simulink model "SimulinkAnalysisofCheetahTail"  (R2022a)
settings: Solver=ode4  StartTime=0.0  StopTime=1.5  FixedStep=0.001  RelTol=1e-3
undefined symbols (not defined in the file): B_cg_H, B_con_H, B_con_L, bar_len, cd_table, Cf, cl_table, g, gear_ratio, int_point_bar, int_point_tail, ITail, M_add, M_cg_H, M_cg_L, M_cg_W, Mb, Mm, Mt, psi3, rho, T_cg_H, T_fur_gap, T_length, T_width_major, T_width_minor, th2_initial, torque_constant, uncertainty_Forces, uncertainty_Position, Vf, windspeed
(part 20 of 21)

== matlab function SimulinkAnalysisofCheetahTail/Model/Forces/NonConstraintForceMatrix_tail_3_added ==
  data: B_con_H parameter; B_con_L parameter; M_add parameter; M_cg_H parameter; M_cg_L parameter; M_cg_W parameter; T_fur_gap parameter; T_length parameter; bar_len parameter; psi3 parameter; Q_added_tail_3_drag output; q input; dq input; ddq input
function Q_added_tail_3_drag = NonConstraintForceMatrix_tail_3_added(B_con_H,B_con_L,M_add,M_cg_H,M_cg_L,M_cg_W,T_fur_gap,T_length,bar_len,psi3,q,dq,ddq)
%#codegen
[x,y,z,phi1,th1,psi1,phi2,th2] = deal(q(1),q(2),q(3),q(4),q(5),q(6),q(7),q(8));
[dx,dy,dz,dphi1,dth1,dpsi1,dphi2,dth2] = deal(dq(1),dq(2),dq(3),dq(4),dq(5),dq(6),dq(7),dq(8));
[ddx,ddy,ddz,ddphi1,ddth1,ddpsi1,ddphi2,ddth2] = deal(ddq(1),ddq(2),ddq(3),ddq(4),ddq(5),ddq(6),ddq(7),ddq(8));
%    This function was generated by the Symbolic Math Toolbox version 9.0.
%    19-Feb-2022 13:43:46

t2 = cos(phi1);
t3 = cos(phi2);
t4 = cos(psi1);
t5 = cos(psi3);
t6 = cos(th1);
t7 = cos(th2);
t8 = sin(phi1);
t9 = sin(phi2);
t10 = sin(psi1);
t11 = sin(psi3);
t12 = sin(th1);
t13 = sin(th2);
t14 = M_cg_L+x;
t15 = M_cg_W+y;
t16 = M_cg_H+z;
t17 = B_con_L.*t6;
t18 = B_con_L.*t12;
t19 = t2.*t4;
t20 = t6.*t7;
t21 = t2.*t10;
t22 = t4.*t8;
t23 = t7.*t12;
t24 = t8.*t10;
t25 = t12.*t13;
t26 = B_con_H.*t2.*t6;
t28 = t6.*t14;
t29 = B_con_H.*t2.*t12;
t30 = B_con_H.*t6.*t8;
t33 = t12.*t14;
t37 = t6.*t9.*t13;
t39 = t6.*t10.*t13;
t41 = t8.*t9.*t12;
t44 = t2.*t3.*t6;
t47 = t2.*t6.*t9;
t48 = t3.*t6.*t8;
t50 = t2.*t6.*t13;
t51 = t3.*t6.*t13;
t53 = t4.*t6.*t13;
t56 = t3.*t8.*t12;
t57 = t6.*t8.*t9;
t62 = t2.*t6.*t15;
t64 = t2.*t6.*t16;
t67 = t6.*t8.*t15;
t68 = t2.*t12.*t16;
t69 = t6.*t8.*t16;
t71 = t8.*t12.*t15;
t99 = t5.*t6.*t8.*t13;
t105 = t6.*t8.*t11.*t13;
t27 = t4.*t17;
t31 = t4.*t18;
t32 = t10.*t17;
t34 = t10.*t18;
t35 = t2.*t25;
t36 = t3.*t25;
t38 = t9.*t23;
t40 = t10.*t23;
t42 = t12.*t24;
t43 = t9.*t25;
t45 = t2.*t20;
t46 = t4.*t20;
t49 = t12.*t19;
t52 = t3.*t23;
t54 = t4.*t23;
t55 = t10.*t20;
t58 = t12.*t21;
t59 = t12.*t22;
t60 = B_con_H.*t6.*t19;
t61 = t4.*t28;
t63 = B_con_H.*t6.*t21;
t65 = t4.*t33;
t66 = t10.*t28;
t70 = t10.*t33;
t72 = -t29;
t73 = -t30;
t75 = -t41;
t80 = t3.*t6.*t22;
t81 = t13.*t44;
t84 = t3.*t8.*t20;
t85 = t6.*t13.*t19;
t86 = t4.*t51;
t89 = t3.*t6.*t24;
t90 = t6.*t9.*t22;
t91 = t2.*t37;
t93 = t8.*t9.*t20;
t94 = t6.*t13.*t21;
t96 = t3.*t39;
t97 = t4.*t37;
t100 = t6.*t9.*t24;
t104 = t10.*t37;
t107 = -t53;
t110 = t6.*t16.*t19;
t111 = t6.*t15.*t22;
t112 = t6.*t16.*t21;
t113 = t6.*t15.*t24;
t114 = -t62;
t115 = -t67;
t116 = -t68;
t117 = -t69;
t118 = t3.*t19.*t20;
t119 = t3.*t20.*t21;
t120 = t9.*t19.*t20;
t121 = t9.*t20.*t21;
t127 = -t99;
t132 = t23+t50;
t74 = -t35;
t76 = -t42;
t77 = -t43;
t78 = t3.*t45;
t79 = t3.*t46;
t82 = t2.*t52;
t83 = t9.*t45;
t87 = t3.*t55;
t88 = t9.*t46;
t92 = t2.*t38;
t95 = t4.*t36;
t98 = t9.*t55;
t101 = -t45;
t102 = t10.*t36;
t103 = t4.*t43;
t106 = -t49;
t108 = -t55;
t109 = t10.*t43;
t123 = -t86;
t125 = -t93;
t130 = -t111;
t131 = -t113;
t133 = t21+t59;
t134 = t22+t58;
t135 = -t118;
t136 = -t119;
t143 = t5.*t132;
t147 = t11.*t132;
t151 = t47+t84;
t155 = t52+t81;
t156 = t54+t85;
t157 = t38+t91;
t158 = t40+t94;
t122 = -t78;
t124 = -t87;
t126 = -t98;
t128 = t4.*t77;
t129 = t10.*t77;
t137 = B_con_H.*t133;
t138 = B_con_H.*t134;
t139 = t20+t74;
t140 = t25+t101;
t141 = t19+t76;
t142 = t24+t106;
t144 = t3.*t133;
t145 = t3.*t134;
t146 = t7.*t134;
t148 = t9.*t133;
t149 = t9.*t134;
t150 = t13.*t134;
t159 = t15.*t133;
t160 = t15.*t134;
t161 = t16.*t133;
t162 = t16.*t134;
t168 = t5.*t13.*t133;
t170 = t11.*t13.*t133;
t178 = -t147;
t182 = t44+t125;
t183 = T_fur_gap.*t151;
t184 = T_fur_gap.*t155;
t185 = bar_len.*t151;
t186 = bar_len.*t155;
t193 = t5.*t156;
t194 = t11.*t156;
t195 = t5.*t157;
t196 = t5.*t158;
t197 = t11.*t157;
t198 = t11.*t158;
t220 = (T_length.*t151)./2.0;
t221 = (T_length.*t155)./2.0;
t223 = t37+t56+t92;
t226 = t51+t75+t82;
t227 = t48+t77+t83;
t264 = t90+t95+t135;
t266 = t100+t102+t136;
t152 = B_con_H.*t141;
t153 = B_con_H.*t142;
t154 = -t138;
t163 = t7.*t144;
t164 = t7.*t145;
t165 = t13.*t145;
t166 = t7.*t148;
t167 = t9.*t146;
t169 = t13.*t149;
t171 = t5.*t139;
t172 = t5.*t140;
t173 = t3.*t141;
t174 = t3.*t142;
t175 = t7.*t142;
t176 = t11.*t139;
t177 = t11.*t140;
t179 = t9.*t141;
t180 = t9.*t142;
t181 = t13.*t142;
t187 = t15.*t141;
t188 = t15.*t142;
t189 = -t160;
t190 = t16.*t141;
t191 = t16.*t142;
t192 = -t162;
t205 = t5.*t13.*t141;
t207 = t11.*t13.*t141;
t208 = -t170;
t214 = t5.*t182;
t215 = t11.*t182;
t216 = -t198;
t222 = t39+t146;
t224 = t108+t150;
t225 = t36+t57+t122;
t231 = t5.*t223;
t232 = t11.*t223;
t235 = T_fur_gap.*t226;
t236 = T_fur_gap.*t227;
t237 = bar_len.*t226;
t238 = bar_len.*t227;
t241 = -t5.*(t55-t150);
t244 = -t11.*(t55-t150);
t245 = t5.*t227;
t247 = t11.*t227;
t257 = (T_length.*t226)./2.0;
t258 = (T_length.*t227)./2.0;
t265 = t80+t120+t128;
t267 = t89+t121+t129;
t274 = T_fur_gap.*t264;
t275 = bar_len.*t264;
t276 = T_fur_gap.*t266;
t277 = bar_len.*t266;
t285 = (T_length.*t264)./2.0;
t286 = (T_length.*t266)./2.0;
t353 = t184+t186+t221;
t373 = t73+t114+t117+t183+t185+t220;
t199 = t7.*t173;
t200 = t7.*t174;
t201 = -t163;
t202 = t13.*t174;
t203 = t7.*t179;
t204 = t9.*t175;
t206 = t13.*t180;
t209 = -t171;
t210 = -t173;
t211 = -t177;
t212 = -t187;
t213 = -t188;
t219 = -t207;
t228 = t46+t181;
t229 = t5.*t222;
t230 = t11.*t222;
t233 = T_fur_gap.*t225;
t234 = bar_len.*t225;
t239 = t107+t175;
t246 = t12.*t225;
t249 = t124+t165;
t251 = t126+t169;
t252 = t2.*t6.*t225;
t253 = -t5.*(t53-t175);
t254 = t6.*t8.*t225;
t255 = -t11.*(t53-t175);
t256 = (T_length.*t225)./2.0;
t261 = -T_fur_gap.*(t87-t165);
t262 = -bar_len.*(t87-t165);
t263 = t105+t214;
t268 = -t5.*(t98-t169);
t270 = -t11.*(t98-t169);
t272 = t5.*(t53-t175);
t278 = t127+t215;
t279 = t5.*t267;
t280 = t11.*t267;
t282 = T_length.*(t87-t165).*(-1.0./2.0);
t283 = t5.*t265;
t284 = t11.*t265;
t288 = t166+t174;
t290 = t172+t197;
t298 = -T_fur_gap.*(t163-t180);
t300 = -bar_len.*(t163-t180);
t303 = T_length.*(t163-t180).*(-1.0./2.0);
t304 = t143+t247;
t305 = t96+t164+t179;
t306 = t176+t231;
t310 = t178+t245;
t328 = -t12.*(t147-t245);
t336 = -t2.*t6.*(t147-t245);
t337 = -t6.*t8.*(t147-t245);
t343 = t2.*t6.*(t147-t245);
t367 = t236+t238+t258;
t368 = t225.*t353;
t385 = -t353.*(t147-t245);
t386 = t353.*(t147-t245);
t388 = -t225.*(t30+t62+t69-t183-t185-t220);
t391 = t17+t28+t71+t72+t116+t235+t237+t257;
t397 = (t147-t245).*(t30+t62+t69-t183-t185-t220);
t407 = t31+t60+t65+t110+t130+t274+t275+t285;
t408 = t34+t63+t70+t112+t131+t276+t277+t286;
t217 = -t199;
t218 = -t204;
t240 = t5.*t228;
t242 = t11.*t228;
t243 = -t229;
t248 = t79+t202;
t250 = t88+t206;
t271 = -t252;
t287 = t145+t203;
t289 = -t283;
t292 = t180+t201;
t294 = t5.*t288;
t296 = t11.*t288;
t301 = t195+t211;
t307 = T_fur_gap.*t305;
t308 = bar_len.*t305;
t309 = t123+t148+t200;
t312 = t209+t232;
t313 = t104+t167+t210;
t314 = t12.*t304;
t321 = (T_length.*t305)./2.0;
t322 = t2.*t6.*t304;
t323 = t6.*t8.*t304;
t324 = t6.*t10.*t305;
t344 = t193+t284;
t345 = t196+t280;
t347 = t216+t279;
t349 = t134.*t305;
t350 = t230+t268;
t355 = t141.*t305;
t383 = t261+t262+t282;
t384 = t304.*t353;
t387 = t225.*t367;
t390 = t18+t26+t33+t64+t115+t233+t234+t256;
t392 = t304.*t367;
t393 = -t304.*(t30+t62+t69-t183-t185-t220);
t395 = -t367.*(t147-t245);
t399 = -t397;
t402 = -t305.*(T_fur_gap.*(t87-t165)+(T_length.*(t87-t165))./2.0+bar_len.*(t87-t165));
t406 = t305.*(T_fur_gap.*(t87-t165)+(T_length.*(t87-t165))./2.0+bar_len.*(t87-t165));
t411 = t225.*t391;
t432 = t304.*t391;
t433 = -t391.*(t147-t245);
t435 = t137+t161+t213+t298+t300+t303;
t441 = t305.*t408;
t259 = T_fur_gap.*t248;
t260 = bar_len.*t248;
t269 = t11.*t250;
t273 = t5.*t250;
t281 = (T_length.*t248)./2.0;
t291 = t149+t217;
t293 = t5.*t287;
t295 = t11.*t287;
t311 = t97+t144+t218;
t315 = T_fur_gap.*t309;
t316 = bar_len.*t309;
t319 = T_fur_gap.*t313;
t320 = bar_len.*t313;
t326 = t5.*t313;
t329 = t11.*t313;
t332 = (T_length.*t309)./2.0;
t334 = (T_length.*t313)./2.0;
t335 = t4.*t6.*t309;
t338 = -t323;
t346 = t194+t289;
t348 = t168+t296;
t351 = t208+t294;
t354 = t133.*t309;
t356 = t243+t270;
t358 = t142.*t309;
t389 = -t387;
t396 = -t392;
t400 = t151.*t390;
t401 = t155.*t390;
t403 = t226.*t390;
t404 = t227.*t390;
t412 = t5.*t225.*t390;
t413 = t11.*t225.*t390;
t417 = t263.*t390;
t419 = -t390.*(t99-t215);
t425 = t290.*t390;
t427 = -t390.*(t177-t195);
t429 = t306.*t390;
t430 = -t390.*(t171-t232);
t434 = -t432;
t442 = -t441;
t443 = t309.*t407;
t447 = t32+t66+t154+t192+t212+t307+t308+t321;
t452 = -t309.*(-t137-t161+t188+T_fur_gap.*(t163-t180)+(T_length.*(t163-t180))./2.0+bar_len.*(t163-t180));
t455 = t309.*(-t137-t161+t188+T_fur_gap.*(t163-t180)+(T_length.*(t163-t180))./2.0+bar_len.*(t163-t180));
t297 = T_fur_gap.*t291;
t299 = bar_len.*t291;
t302 = (T_length.*t291)./2.0;
t317 = T_fur_gap.*t311;
t318 = bar_len.*t311;
t325 = t5.*t311;
t327 = t11.*t311;
t330 = -t315;
t331 = -t316;
t333 = (T_length.*t311)./2.0;
t339 = -t326;
t341 = -t332;
t342 = -t335;
t352 = t205+t295;
t357 = t219+t293;
t359 = t255+t273;
t360 = t269+t272;
t362 = t241+t329;
t366 = t6.*t10.*(t329-t5.*(t55-t150));
t371 = -t6.*t10.*(t326+t11.*(t55-t150));
t375 = t134.*(t329-t5.*(t55-t150));
t378 = t141.*(t329-t5.*(t55-t150));
t379 = -t134.*(t326+t11.*(t55-t150));
t381 = -t141.*(t326+t11.*(t55-t150));
t382 = t259+t260+t281;
t409 = -t404;
t414 = -t412;
t415 = t319+t320+t334;
t418 = t254+t354+t355;
t420 = -t417;
t422 = t271+t349+t358;
t428 = -t425;
t431 = -t429;
t438 = -(t329-t5.*(t55-t150)).*(T_fur_gap.*(t87-t165)+(T_length.*(t87-t165))./2.0+bar_len.*(t87-t165));
t440 = (t326+t11.*(t55-t150)).*(T_fur_gap.*(t87-t165)+(T_length.*(t87-t165))./2.0+bar_len.*(t87-t165));
t458 = t408.*(t329-t5.*(t55-t150));
t460 = -t408.*(t326+t11.*(t55-t150));
t464 = t408.*(t326+t11.*(t55-t150));
t477 = -t447.*(t87-t165);
t478 = t447.*(t87-t165);
t479 = t266.*t447;
t484 = t291.*t447;
t492 = t5.*t305.*t447;
t493 = t11.*t305.*t447;
t494 = t313.*t447;
t497 = t345.*t447;
t500 = -t447.*(t198-t279);
t502 = t447.*(t198-t279);
t503 = t350.*t447;
t506 = -t447.*(t229+t11.*(t98-t169));
t508 = -t447.*(t207-t293);
t340 = -t327;
t361 = t242+t325;
t364 = t244+t339;
t372 = -t366;
t394 = t246+t324+t342;
t405 = t309.*t382;
t416 = t317+t318+t333;
t421 = ddy.*t418;
t423 = ddz.*t422;
t437 = t152+t189+t190+t297+t299+t302;
t444 = t305.*t415;
t448 = t27+t61+t153+t159+t191+t330+t331+t341;
t461 = -t458;
t465 = t415.*(t329-t5.*(t55-t150));
t467 = -t415.*(t326+t11.*(t55-t150));
t469 = t415.*(t326+t11.*(t55-t150));
t481 = -t479;
t486 = -t484;
t495 = -t492;
t504 = t352.*t447;
t507 = -t503;
t363 = t240+t340;
t365 = t4.*t6.*t361;
t374 = t133.*t361;
t376 = t142.*t361;
t398 = ddx.*t394;
t410 = -t405;
t424 = -t421;
t426 = -t423;
t436 = t361.*t382;
t445 = t309.*t416;
t453 = t305.*t437;
t459 = t361.*t407;
t463 = t361.*t416;
t468 = -t465;
t482 = t248.*t448;
t483 = t264.*t448;
t487 = -t361.*(-t137-t161+t188+T_fur_gap.*(t163-t180)+(T_length.*(t163-t180))./2.0+bar_len.*(t163-t180));
t489 = t437.*(t329-t5.*(t55-t150));
t490 = -t437.*(t326+t11.*(t55-t150));
t491 = -t448.*(t163-t180);
t496 = t311.*t448;
t498 = t5.*t309.*t448;
t499 = t11.*t309.*t448;
t505 = t344.*t448;
t509 = -t504;
t510 = t346.*t448;
t511 = t348.*t448;
t512 = -t448.*(t170-t294);
t513 = t448.*(t170-t294);
t514 = t359.*t448;
t515 = t360.*t448;
t369 = t4.*t6.*t363;
t370 = -t365;
t377 = t133.*t363;
t380 = t142.*t363;
t439 = t363.*t382;
t446 = -t445;
t454 = -ddx.*(t365+t12.*(t147-t245)+t6.*t10.*(t326+t11.*(t55-t150)));
t456 = -t453;
t457 = ddx.*(t365+t12.*(t147-t245)+t6.*t10.*(t326+t11.*(t55-t150)));
t462 = t363.*t407;
t466 = t363.*t416;
Q_added_tail_3_drag = ft_1({M_add,T_fur_gap,T_length,bar_len,ddphi1,ddphi2,ddth1,ddth2,ddx,ddy,ddz,t10,t11,t12,t132,t133,t134,t137,t141,t142,t147,t150,t161,t163,t165,t169,t171,t180,t183,t185,t188,t2,t207,t215,t220,t225,t227,t228,t229,t232,t245,t293,t30,t304,t305,t309,t311,t313,t314,t322,t326,t328,t329,t337,t338,t343,t353,t361,t363,t367,t368,t369,t370,t371,t372,t374,t375,t376,t377,t378,t379,t380,t381,t382,t384,t386,t387,t388,t389,t390,t391,t392,t393,t395,t396,t397,t398,t399,t4,t400,t401,t403,t404,t406,t407,t408,t409,t410,t411,t413,t414,t415,t416,t417,t419,t420,t424,t425,t426,t427,t428,t430,t431,t432,t433,t434,t436,t437,t438,t439,t440,t442,t443,t444,t445,t446,t447,t448,t452,t453,t454,t455,t456,t457,t458,t459,t461,t462,t463,t464,t465,t466,t468,t469,t478,t481,t482,t483,t484,t486,t487,t489,t490,t491,t493,t494,t495,t496,t497,t498,t499,t5,t502,t504,t505,t506,t507,t508,t509,t510,t511,t512,t513,t514,t515,t55,t6,t62,t69,t8,t87,t98,t99});
end
function Q_added_tail_3_drag = ft_1(ct)
M_add = ct{1};
T_fur_gap = ct{2};
T_length = ct{3};
bar_len = ct{4};
ddphi1 = ct{5};
ddphi2 = ct{6};
ddth1 = ct{7};
ddth2 = ct{8};
ddx = ct{9};
ddy = ct{10};
ddz = ct{11};
t10 = ct{12};
t11 = ct{13};
t12 = ct{14};
t132 = ct{15};
t133 = ct{16};
t134 = ct{17};
t137 = ct{18};
t141 = ct{19};
t142 = ct{20};
t147 = ct{21};
t150 = ct{22};
t161 = ct{23};
t163 = ct{24};
t165 = ct{25};
t169 = ct{26};
t171 = ct{27};
t180 = ct{28};
t183 = ct{29};
t185 = ct{30};
t188 = ct{31};
t2 = ct{32};
t207 = ct{33};
t215 = ct{34};
t220 = ct{35};
t225 = ct{36};
t227 = ct{37};
t228 = ct{38};
t229 = ct{39};
t232 = ct{40};
t245 = ct{41};
t293 = ct{42};
t30 = ct{43};
t304 = ct{44};
t305 = ct{45};
t309 = ct{46};
t311 = ct{47};
t313 = ct{48};
t314 = ct{49};
t322 = ct{50};
t326 = ct{51};
t328 = ct{52};
t329 = ct{53};
t337 = ct{54};
t338 = ct{55};
t343 = ct{56};
t353 = ct{57};
t361 = ct{58};
t363 = ct{59};
t367 = ct{60};
t368 = ct{61};
t369 = ct{62};
t370 = ct{63};
t371 = ct{64};
t372 = ct{65};
t374 = ct{66};
t375 = ct{67};
t376 = ct{68};
t377 = ct{69};
t378 = ct{70};
t379 = ct{71};
t380 = ct{72};
t381 = ct{73};
t382 = ct{74};
t384 = ct{75};
t386 = ct{76};
t387 = ct{77};
t388 = ct{78};
t389 = ct{79};
t390 = ct{80};
t391 = ct{81};
t392 = ct{82};
t393 = ct{83};
t395 = ct{84};
t396 = ct{85};
t397 = ct{86};
t398 = ct{87};
t399 = ct{88};
t4 = ct{89};
t400 = ct{90};
t401 = ct{91};
t403 = ct{92};
t404 = ct{93};
t406 = ct{94};
t407 = ct{95};
t408 = ct{96};
t409 = ct{97};
t410 = ct{98};
t411 = ct{99};
t413 = ct{100};
t414 = ct{101};
t415 = ct{102};
t416 = ct{103};
t417 = ct{104};
t419 = ct{105};
t420 = ct{106};
t424 = ct{107};
t425 = ct{108};
t426 = ct{109};
t427 = ct{110};
t428 = ct{111};
t430 = ct{112};
t431 = ct{113};
t432 = ct{114};
t433 = ct{115};
t434 = ct{116};
t436 = ct{117};
t437 = ct{118};
t438 = ct{119};
t439 = ct{120};
t440 = ct{121};
t442 = ct{122};
t443 = ct{123};
t444 = ct{124};
t445 = ct{125};
t446 = ct{126};
t447 = ct{127};
t448 = ct{128};
t452 = ct{129};
t453 = ct{130};
t454 = ct{131};
t455 = ct{132};
t456 = ct{133};
t457 = ct{134};
t458 = ct{135};
t459 = ct{136};
t461 = ct{137};
t462 = ct{138};
t463 = ct{139};
t464 = ct{140};
t465 = ct{141};
t466 = ct{142};
t468 = ct{143};
t469 = ct{144};
t478 = ct{145};
t481 = ct{146};
t482 = ct{147};
t483 = ct{148};
t484 = ct{149};
t486 = ct{150};
t487 = ct{151};
t489 = ct{152};
t490 = ct{153};
t491 = ct{154};
t493 = ct{155};
t494 = ct{156};
t495 = ct{157};
t496 = ct{158};
t497 = ct{159};
t498 = ct{160};
t499 = ct{161};
t5 = ct{162};
t502 = ct{163};
t504 = ct{164};
t505 = ct{165};
t506 = ct{166};
t507 = ct{167};
t508 = ct{168};
t509 = ct{169};
t510 = ct{170};
t511 = ct{171};
t512 = ct{172};
t513 = ct{173};
t514 = ct{174};
t515 = ct{175};
t55 = ct{176};
t6 = ct{177};
t62 = ct{178};
t69 = ct{179};
t8 = ct{180};
t87 = ct{181};
t98 = ct{182};
t99 = ct{183};
t471 = t337+t374+t381;
t474 = -ddy.*(-t374+t141.*(t326+t11.*(t55-t150))+t6.*t8.*(t147-t245));
t476 = t343+t376+t379;
t485 = -t483;
t488 = -t363.*(-t137-t161+t188+T_fur_gap.*(t163-t180)+(T_length.*(t163-t180))./2.0+bar_len.*(t163-t180));
t501 = -t499;
t516 = -t515;
t517 = t368+t401+t406+t410+t478+t482;
t522 = t386+t427+t436+t440+t507+t514;
t524 = -ddphi2.*(t387+t404-t444+t445-t494-t496);
t527 = ddphi2.*(t387+t404-t444+t445-t494-t496);
t529 = -ddphi1.*(-t400+t452+t453+t484+t225.*(t30+t62+t69-t183-t185-t220)+t448.*(t163-t180));
t532 = t395+t414+t463+t469+t495+t498;
t539 = t431+t433+t459+t464+t502+t510;
t543 = -ddphi1.*(-t489+t504-t511+t304.*(t30+t62+t69-t183-t185-t220)+t363.*(-t137-t161+t188+T_fur_gap.*(t163-t180)+(T_length.*(t163-t180))./2.0+bar_len.*(t163-t180))+t390.*(t99-t215));
t544 = t399+t420+t487+t490+t508+t513;
t545 = -ddphi1.*(t397+t417+t512+t437.*(t326+t11.*(t55-t150))+t361.*(-t137-t161+t188+T_fur_gap.*(t163-t180)+(T_length.*(t163-t180))./2.0+bar_len.*(t163-t180))+t447.*(t207-t293));
t449 = t314+t369+t372;
t451 = t328+t370+t371;
t470 = t322+t375+t380;
t472 = t338+t377+t378;
t480 = ddz.*t476;
t518 = ddth2.*t517;
t519 = t403+t411+t442+t443+t481+t485;
t521 = t389+t409+t444+t446+t494+t496;
t523 = t384+t428+t438+t439+t506+t516;
t525 = ddth2.*t522;
t526 = -ddth2.*(-t384+t425-t439+t515+t447.*(t229+t11.*(t98-t169))+(t329-t5.*(t55-t150)).*(T_fur_gap.*(t87-t165)+(T_length.*(t87-t165))./2.0+bar_len.*(t87-t165)));
t528 = t388+t400+t455+t456+t486+t491;
t530 = t396+t413+t466+t468+t493+t501;
t531 = -ddphi2.*(t392-t413+t465-t466-t493+t499);
t533 = ddphi2.*(t392-t413+t465-t466-t493+t499);
t534 = ddphi2.*t532;
t536 = t430+t434+t461+t462+t497+t505;
t537 = -ddth1.*(t432+t458-t462-t497-t505+t390.*(t171-t232));
t538 = ddth1.*(t432+t458-t462-t497-t505+t390.*(t171-t232));
t540 = ddth1.*t539;
t542 = t393+t419+t488+t489+t509+t511;
t450 = ddx.*t449;
t473 = ddz.*t470;
t475 = ddy.*t472;
t520 = ddth1.*t519;
t535 = -t534;
t541 = -t540;
t557 = -M_add.*t227.*(t454-t480-t525+t534+t540+ddy.*(-t374+t141.*(t326+t11.*(t55-t150))+t6.*t8.*(t147-t245))+ddphi1.*(t397+t417+t512+t437.*(t326+t11.*(t55-t150))+t361.*(-t137-t161+t188+T_fur_gap.*(t163-t180)+(T_length.*(t163-t180))./2.0+bar_len.*(t163-t180))+t447.*(t207-t293)));
t558 = M_add.*t227.*(t454-t480-t525+t534+t540+ddy.*(-t374+t141.*(t326+t11.*(t55-t150))+t6.*t8.*(t147-t245))+ddphi1.*(t397+t417+t512+t437.*(t326+t11.*(t55-t150))+t361.*(-t137-t161+t188+T_fur_gap.*(t163-t180)+(T_length.*(t163-t180))./2.0+bar_len.*(t163-t180))+t447.*(t207-t293)));
t559 = -M_add.*t311.*(t454-t480-t525+t534+t540+ddy.*(-t374+t141.*(t326+t11.*(t55-t150))+t6.*t8.*(t147-t245))+ddphi1.*(t397+t417+t512+t437.*(t326+t11.*(t55-t150))+t361.*(-t137-t161+t188+T_fur_gap.*(t163-t180)+(T_length.*(t163-t180))./2.0+bar_len.*(t163-t180))+t447.*(t207-t293)));
t560 = -M_add.*t313.*(t454-t480-t525+t534+t540+ddy.*(-t374+t141.*(t326+t11.*(t55-t150))+t6.*t8.*(t147-t245))+ddphi1.*(t397+t417+t512+t437.*(t326+t11.*(t55-t150))+t361.*(-t137-t161+t188+T_fur_gap.*(t163-t180)+(T_length.*(t163-t180))./2.0+bar_len.*(t163-t180))+t447.*(t207-t293)));
t546 = t398+t424+t426+t518+t520+t527+t529;
t551 = t450+t473+t475+t526+t533+t538+t543;
t553 = t457+t474+t480+t525+t535+t541+t545;
t547 = M_add.*t225.*t546;
t548 = M_add.*t305.*t546;
t549 = M_add.*t309.*t546;
t552 = M_add.*t132.*t551;
t554 = M_add.*t228.*t551;
t555 = -M_add.*t551.*(t55-t150);
t556 = M_add.*t551.*(t55-t150);
t550 = -t549;
t561 = t547+t552+t558;
t562 = t548+t556+t560;
t563 = t550+t554+t559;
mt1 = [-t12.*t561-t6.*t10.*t562+t4.*t6.*(t549-t554+M_add.*t311.*(t454-t480-t525+t534+t540+ddy.*(-t374+t141.*(t326+t11.*(t55-t150))+t6.*t8.*(t147-t245))+ddphi1.*(t397+t417+t512+t437.*(t326+t11.*(t55-t150))+t361.*(-t137-t161+t188+T_fur_gap.*(t163-t180)+(T_length.*(t163-t180))./2.0+bar_len.*(t163-t180))+t447.*(t207-t293))))];
mt2 = [t141.*t562+t133.*(t549-t554+M_add.*t311.*(t454-t480-t525+t534+t540+ddy.*(-t374+t141.*(t326+t11.*(t55-t150))+t6.*t8.*(t147-t245))+ddphi1.*(t397+t417+t512+t437.*(t326+t11.*(t55-t150))+t361.*(-t137-t161+t188+T_fur_gap.*(t163-t180)+(T_length.*(t163-t180))./2.0+bar_len.*(t163-t180))+t447.*(t207-t293))))+t6.*t8.*t561];
mt3 = [t134.*t562+t142.*(t549-t554+M_add.*t311.*(t454-t480-t525+t534+t540+ddy.*(-t374+t141.*(t326+t11.*(t55-t150))+t6.*t8.*(t147-t245))+ddphi1.*(t397+t417+t512+t437.*(t326+t11.*(t55-t150))+t361.*(-t137-t161+t188+T_fur_gap.*(t163-t180)+(T_length.*(t163-t180))./2.0+bar_len.*(t163-t180))+t447.*(t207-t293))))-t2.*t6.*t561];
mt4 = [t561.*(t30+t62+t69-t183-t185-t220)+t437.*t562-(t549-t554+M_add.*t311.*(t454-t480-t525+t534+t540+ddy.*(-t374+t141.*(t326+t11.*(t55-t150))+t6.*t8.*(t147-t245))+ddphi1.*(t397+t417+t512+t437.*(t326+t11.*(t55-t150))+t361.*(-t137-t161+t188+T_fur_gap.*(t163-t180)+(T_length.*(t163-t180))./2.0+bar_len.*(t163-t180))+t447.*(t207-t293)))).*(-t137-t161+t188+T_fur_gap.*(t163-t180)+(T_length.*(t163-t180))./2.0+bar_len.*(t163-t180))];
mt5 = [-t391.*t561+t408.*t562-t407.*(t549-t554+M_add.*t311.*(t454-t480-t525+t534+t540+ddy.*(-t374+t141.*(t326+t11.*(t55-t150))+t6.*t8.*(t147-t245))+ddphi1.*(t397+t417+t512+t437.*(t326+t11.*(t55-t150))+t361.*(-t137-t161+t188+T_fur_gap.*(t163-t180)+(T_length.*(t163-t180))./2.0+bar_len.*(t163-t180))+t447.*(t207-t293))))];
mt6 = [-t448.*t562-t447.*(t549-t554+M_add.*t311.*(t454-t480-t525+t534+t540+ddy.*(-t374+t141.*(t326+t11.*(t55-t150))+t6.*t8.*(t147-t245))+ddphi1.*(t397+t417+t512+t437.*(t326+t11.*(t55-t150))+t361.*(-t137-t161+t188+T_fur_gap.*(t163-t180)+(T_length.*(t163-t180))./2.0+bar_len.*(t163-t180))+t447.*(t207-t293))))];
mt7 = [-t367.*t561+t415.*t562-t416.*(t549-t554+M_add.*t311.*(t454-t480-t525+t534+t540+ddy.*(-t374+t141.*(t326+t11.*(t55-t150))+t6.*t8.*(t147-t245))+ddphi1.*(t397+t417+t512+t437.*(t326+t11.*(t55-t150))+t361.*(-t137-t161+t188+T_fur_gap.*(t163-t180)+(T_length.*(t163-t180))./2.0+bar_len.*(t163-t180))+t447.*(t207-t293))))];
mt8 = [-t353.*t561-t562.*(T_fur_gap.*(t87-t165)+(T_length.*(t87-t165))./2.0+bar_len.*(t87-t165))+t382.*(t549-t554+M_add.*t311.*(t454-t480-t525+t534+t540+ddy.*(-t374+t141.*(t326+t11.*(t55-t150))+t6.*t8.*(t147-t245))+ddphi1.*(t397+t417+t512+t437.*(t326+t11.*(t55-t150))+t361.*(-t137-t161+t188+T_fur_gap.*(t163-t180)+(T_length.*(t163-t180))./2.0+bar_len.*(t163-t180))+t447.*(t207-t293))))];
Q_added_tail_3_drag = [mt1;mt2;mt3;mt4;mt5;mt6;mt7;mt8];
end

== matlab function SimulinkAnalysisofCheetahTail/Model/Forces/NonConstraintForceMatrix_tail_4_added ==
  data: B_con_H parameter; B_con_L parameter; M_add parameter; M_cg_H parameter; M_cg_L parameter; M_cg_W parameter; T_fur_gap parameter; T_length parameter; bar_len parameter; psi3 parameter; Q_added_tail_4_drag output; q input; dq input; ddq input
function Q_added_tail_4_drag = NonConstraintForceMatrix_tail_4_added(B_con_H,B_con_L,M_add,M_cg_H,M_cg_L,M_cg_W,T_fur_gap,T_length,bar_len,psi3,q,dq,ddq)
%#codegen
[x,y,z,phi1,th1,psi1,phi2,th2] = deal(q(1),q(2),q(3),q(4),q(5),q(6),q(7),q(8));
[dx,dy,dz,dphi1,dth1,dpsi1,dphi2,dth2] = deal(dq(1),dq(2),dq(3),dq(4),dq(5),dq(6),dq(7),dq(8));
[ddx,ddy,ddz,ddphi1,ddth1,ddpsi1,ddphi2,ddth2] = deal(ddq(1),ddq(2),ddq(3),ddq(4),ddq(5),ddq(6),ddq(7),ddq(8));
%    This function was generated by the Symbolic Math Toolbox version 9.0.
%    19-Feb-2022 13:44:13

t2 = cos(phi1);
t3 = cos(phi2);
t4 = cos(psi1);
t5 = cos(psi3);
t6 = cos(th1);
t7 = cos(th2);
t8 = sin(phi1);
t9 = sin(phi2);
t10 = sin(psi1);
t11 = sin(psi3);
t12 = sin(th1);
t13 = sin(th2);
t14 = M_cg_L+x;
t15 = M_cg_W+y;
t16 = M_cg_H+z;
t17 = B_con_L.*t6;
t18 = B_con_L.*t12;
t19 = t2.*t4;
t20 = t6.*t7;
t21 = t2.*t10;
t22 = t4.*t8;
t23 = t7.*t12;
t24 = t8.*t10;
t25 = t12.*t13;
t26 = B_con_H.*t2.*t6;
t28 = t6.*t14;
t29 = B_con_H.*t2.*t12;
t30 = B_con_H.*t6.*t8;
t33 = t12.*t14;
t37 = t6.*t9.*t13;
t39 = t6.*t10.*t13;
t41 = t8.*t9.*t12;
t44 = t2.*t3.*t6;
t47 = t2.*t6.*t9;
t48 = t3.*t6.*t8;
t50 = t2.*t6.*t13;
t51 = t3.*t6.*t13;
t53 = t4.*t6.*t13;
t56 = t3.*t8.*t12;
t57 = t6.*t8.*t9;
t62 = t2.*t6.*t15;
t64 = t2.*t6.*t16;
t67 = t6.*t8.*t15;
t68 = t2.*t12.*t16;
t69 = t6.*t8.*t16;
t71 = t8.*t12.*t15;
t99 = t5.*t6.*t8.*t13;
t105 = t6.*t8.*t11.*t13;
t27 = t4.*t17;
t31 = t4.*t18;
t32 = t10.*t17;
t34 = t10.*t18;
t35 = t2.*t25;
t36 = t3.*t25;
t38 = t9.*t23;
t40 = t10.*t23;
t42 = t12.*t24;
t43 = t9.*t25;
t45 = t2.*t20;
t46 = t4.*t20;
t49 = t12.*t19;
t52 = t3.*t23;
t54 = t4.*t23;
t55 = t10.*t20;
t58 = t12.*t21;
t59 = t12.*t22;
t60 = B_con_H.*t6.*t19;
t61 = t4.*t28;
t63 = B_con_H.*t6.*t21;
t65 = t4.*t33;
t66 = t10.*t28;
t70 = t10.*t33;
t72 = -t29;
t73 = -t30;
t75 = -t41;
t80 = t3.*t6.*t22;
t81 = t13.*t44;
t84 = t3.*t8.*t20;
t85 = t6.*t13.*t19;
t86 = t4.*t51;
t89 = t3.*t6.*t24;
t90 = t6.*t9.*t22;
t91 = t2.*t37;
t93 = t8.*t9.*t20;
t94 = t6.*t13.*t21;
t96 = t3.*t39;
t97 = t4.*t37;
t100 = t6.*t9.*t24;
t104 = t10.*t37;
t107 = -t53;
t110 = t6.*t16.*t19;
t111 = t6.*t15.*t22;
t112 = t6.*t16.*t21;
t113 = t6.*t15.*t24;
t114 = -t62;
t115 = -t67;
t116 = -t68;
t117 = -t69;
t118 = t3.*t19.*t20;
t119 = t3.*t20.*t21;
t120 = t9.*t19.*t20;
t121 = t9.*t20.*t21;
t127 = -t99;
t132 = t23+t50;
t74 = -t35;
t76 = -t42;
t77 = -t43;
t78 = t3.*t45;
t79 = t3.*t46;
t82 = t2.*t52;
t83 = t9.*t45;
t87 = t3.*t55;
t88 = t9.*t46;
t92 = t2.*t38;
t95 = t4.*t36;
t98 = t9.*t55;
t101 = -t45;
t102 = t10.*t36;
t103 = t4.*t43;
t106 = -t49;
t108 = -t55;
t109 = t10.*t43;
t123 = -t86;
t125 = -t93;
t130 = -t111;
t131 = -t113;
t133 = t21+t59;
t134 = t22+t58;
t135 = -t118;
t136 = -t119;
t143 = t5.*t132;
t147 = t11.*t132;
t151 = t47+t84;
t155 = t52+t81;
t156 = t54+t85;
t157 = t38+t91;
t158 = t40+t94;
t122 = -t78;
t124 = -t87;
t126 = -t98;
t128 = t4.*t77;
t129 = t10.*t77;
t137 = B_con_H.*t133;
t138 = B_con_H.*t134;
t139 = t20+t74;
t140 = t25+t101;
t141 = t19+t76;
t142 = t24+t106;
t144 = t3.*t133;
t145 = t3.*t134;
t146 = t7.*t134;
t148 = t9.*t133;
t149 = t9.*t134;
t150 = t13.*t134;
t159 = t15.*t133;
t160 = t15.*t134;
t161 = t16.*t133;
t162 = t16.*t134;
t168 = t5.*t13.*t133;
t170 = t11.*t13.*t133;
t178 = -t147;
t182 = t44+t125;
t183 = T_fur_gap.*t151;
t184 = T_fur_gap.*t155;
t185 = bar_len.*t151;
t186 = bar_len.*t155;
t193 = t5.*t156;
t194 = t11.*t156;
t195 = t5.*t157;
t196 = t5.*t158;
t197 = t11.*t157;
t198 = t11.*t158;
t220 = T_length.*t151.*(7.0./1.0e+1);
t221 = T_length.*t155.*(7.0./1.0e+1);
t223 = t37+t56+t92;
t226 = t51+t75+t82;
t227 = t48+t77+t83;
t261 = t90+t95+t135;
t263 = t100+t102+t136;
t152 = B_con_H.*t141;
t153 = B_con_H.*t142;
t154 = -t138;
t163 = t7.*t144;
t164 = t7.*t145;
t165 = t13.*t145;
t166 = t7.*t148;
t167 = t9.*t146;
t169 = t13.*t149;
t171 = t5.*t139;
t172 = t5.*t140;
t173 = t3.*t141;
t174 = t3.*t142;
t175 = t7.*t142;
t176 = t11.*t139;
t177 = t11.*t140;
t179 = t9.*t141;
t180 = t9.*t142;
t181 = t13.*t142;
t187 = t15.*t141;
t188 = t15.*t142;
t189 = -t160;
t190 = t16.*t141;
t191 = t16.*t142;
t192 = -t162;
t205 = t5.*t13.*t141;
t207 = t11.*t13.*t141;
t208 = -t170;
t214 = t5.*t182;
t215 = t11.*t182;
t216 = -t198;
t222 = t39+t146;
t224 = t108+t150;
t225 = t36+t57+t122;
t231 = t5.*t223;
t232 = t11.*t223;
t235 = T_fur_gap.*t226;
t236 = T_fur_gap.*t227;
t237 = bar_len.*t226;
t238 = bar_len.*t227;
t241 = -t5.*(t55-t150);
t244 = -t11.*(t55-t150);
t245 = t5.*t227;
t247 = t11.*t227;
t262 = t80+t120+t128;
t265 = t89+t121+t129;
t266 = T_length.*t226.*(7.0./1.0e+1);
t267 = T_length.*t227.*(7.0./1.0e+1);
t274 = T_fur_gap.*t261;
t275 = bar_len.*t261;
t276 = T_fur_gap.*t263;
t277 = bar_len.*t263;
t288 = T_length.*t261.*(7.0./1.0e+1);
t289 = T_length.*t263.*(7.0./1.0e+1);
t355 = t184+t186+t221;
t373 = t73+t114+t117+t183+t185+t220;
t199 = t7.*t173;
t200 = t7.*t174;
t201 = -t163;
t202 = t13.*t174;
t203 = t7.*t179;
t204 = t9.*t175;
t206 = t13.*t180;
t209 = -t171;
t210 = -t173;
t211 = -t177;
t212 = -t187;
t213 = -t188;
t219 = -t207;
t228 = t46+t181;
t229 = t5.*t222;
t230 = t11.*t222;
t233 = T_fur_gap.*t225;
t234 = bar_len.*t225;
t239 = t107+t175;
t246 = t12.*t225;
t249 = t124+t165;
t251 = t126+t169;
t252 = t2.*t6.*t225;
t253 = -t5.*(t53-t175);
t254 = t6.*t8.*t225;
t255 = -t11.*(t53-t175);
t258 = -T_fur_gap.*(t87-t165);
t259 = -bar_len.*(t87-t165);
t260 = t105+t214;
t264 = T_length.*t225.*(7.0./1.0e+1);
t268 = -t5.*(t98-t169);
t270 = -t11.*(t98-t169);
t272 = t5.*(t53-t175);
t278 = t127+t215;
t279 = t5.*t265;
t280 = t11.*t265;
t281 = t5.*t262;
t282 = t11.*t262;
t284 = T_length.*(t87-t165).*(-7.0./1.0e+1);
t286 = t166+t174;
t290 = t172+t197;
t298 = -T_fur_gap.*(t163-t180);
t300 = -bar_len.*(t163-t180);
t303 = T_length.*(t163-t180).*(-7.0./1.0e+1);
t304 = t143+t247;
t305 = t96+t164+t179;
t306 = t176+t231;
t310 = t178+t245;
t327 = -t12.*(t147-t245);
t333 = -t2.*t6.*(t147-t245);
t334 = -t6.*t8.*(t147-t245);
t343 = t2.*t6.*(t147-t245);
t371 = t236+t238+t267;
t372 = t225.*t355;
t385 = -t355.*(t147-t245);
t386 = t355.*(t147-t245);
t388 = -t225.*(t30+t62+t69-t183-t185-t220);
t391 = t17+t28+t71+t72+t116+t235+t237+t266;
t398 = (t147-t245).*(t30+t62+t69-t183-t185-t220);
t407 = t31+t60+t65+t110+t130+t274+t275+t288;
t408 = t34+t63+t70+t112+t131+t276+t277+t289;
t217 = -t199;
t218 = -t204;
t240 = t5.*t228;
t242 = t11.*t228;
t243 = -t229;
t248 = t79+t202;
t250 = t88+t206;
t271 = -t252;
t285 = t145+t203;
t287 = -t281;
t292 = t180+t201;
t294 = t5.*t286;
t296 = t11.*t286;
t301 = t195+t211;
t307 = T_fur_gap.*t305;
t308 = bar_len.*t305;
t309 = t123+t148+t200;
t312 = t209+t232;
t313 = t104+t167+t210;
t314 = t12.*t304;
t321 = t2.*t6.*t304;
t322 = t6.*t8.*t304;
t323 = t6.*t10.*t305;
t331 = T_length.*t305.*(7.0./1.0e+1);
t344 = t193+t282;
t345 = t196+t280;
t347 = t216+t279;
t349 = t134.*t305;
t350 = t230+t268;
t354 = t141.*t305;
t383 = t258+t259+t284;
t384 = t304.*t355;
t387 = t225.*t371;
t390 = t18+t26+t33+t64+t115+t233+t234+t264;
t393 = t304.*t371;
t394 = -t304.*(t30+t62+t69-t183-t185-t220);
t396 = -t371.*(t147-t245);
t399 = -t398;
t402 = -t305.*(T_fur_gap.*(t87-t165)+T_length.*(t87-t165).*(7.0./1.0e+1)+bar_len.*(t87-t165));
t406 = t305.*(T_fur_gap.*(t87-t165)+T_length.*(t87-t165).*(7.0./1.0e+1)+bar_len.*(t87-t165));
t411 = t225.*t391;
t432 = t304.*t391;
t433 = -t391.*(t147-t245);
t435 = t137+t161+t213+t298+t300+t303;
t441 = t305.*t408;
t256 = T_fur_gap.*t248;
t257 = bar_len.*t248;
t269 = t11.*t250;
t273 = t5.*t250;
t283 = T_length.*t248.*(7.0./1.0e+1);
t291 = t149+t217;
t293 = t5.*t285;
t295 = t11.*t285;
t311 = t97+t144+t218;
t315 = T_fur_gap.*t309;
t316 = bar_len.*t309;
t319 = T_fur_gap.*t313;
t320 = bar_len.*t313;
t325 = t5.*t313;
t328 = t11.*t313;
t332 = t4.*t6.*t309;
t335 = -t322;
t338 = T_length.*t309.*(7.0./1.0e+1);
t340 = T_length.*t313.*(7.0./1.0e+1);
t346 = t194+t287;
t348 = t168+t296;
t351 = t208+t294;
t353 = t133.*t309;
t356 = t243+t270;
t358 = t142.*t309;
t389 = -t387;
t397 = -t393;
t400 = t151.*t390;
t401 = t155.*t390;
t403 = t226.*t390;
t404 = t227.*t390;
t412 = t5.*t225.*t390;
t413 = t11.*t225.*t390;
t418 = t260.*t390;
t419 = -t390.*(t99-t215);
t426 = t290.*t390;
t427 = -t390.*(t177-t195);
t429 = t306.*t390;
t430 = -t390.*(t171-t232);
t434 = -t432;
t442 = -t441;
t443 = t309.*t407;
t447 = t32+t66+t154+t192+t212+t307+t308+t331;
t452 = -t309.*(-t137-t161+t188+T_fur_gap.*(t163-t180)+T_length.*(t163-t180).*(7.0./1.0e+1)+bar_len.*(t163-t180));
t455 = t309.*(-t137-t161+t188+T_fur_gap.*(t163-t180)+T_length.*(t163-t180).*(7.0./1.0e+1)+bar_len.*(t163-t180));
t297 = T_fur_gap.*t291;
t299 = bar_len.*t291;
t302 = T_length.*t291.*(7.0./1.0e+1);
t317 = T_fur_gap.*t311;
t318 = bar_len.*t311;
t324 = t5.*t311;
t326 = t11.*t311;
t329 = -t315;
t330 = -t316;
t336 = -t325;
t339 = T_length.*t311.*(7.0./1.0e+1);
t341 = -t338;
t342 = -t332;
t352 = t205+t295;
t357 = t219+t293;
t359 = t255+t273;
t360 = t269+t272;
t362 = t241+t328;
t366 = t6.*t10.*(t328-t5.*(t55-t150));
t369 = -t6.*t10.*(t325+t11.*(t55-t150));
t375 = t134.*(t328-t5.*(t55-t150));
t378 = t141.*(t328-t5.*(t55-t150));
t379 = -t134.*(t325+t11.*(t55-t150));
t381 = -t141.*(t325+t11.*(t55-t150));
t382 = t256+t257+t283;
t409 = -t404;
t414 = -t412;
t415 = t319+t320+t340;
t417 = t254+t353+t354;
t420 = -t418;
t422 = t271+t349+t358;
t428 = -t426;
t431 = -t429;
t438 = -(t328-t5.*(t55-t150)).*(T_fur_gap.*(t87-t165)+T_length.*(t87-t165).*(7.0./1.0e+1)+bar_len.*(t87-t165));
t440 = (t325+t11.*(t55-t150)).*(T_fur_gap.*(t87-t165)+T_length.*(t87-t165).*(7.0./1.0e+1)+bar_len.*(t87-t165));
t458 = t408.*(t328-t5.*(t55-t150));
t460 = -t408.*(t325+t11.*(t55-t150));
t464 = t408.*(t325+t11.*(t55-t150));
t477 = -t447.*(t87-t165);
t479 = t447.*(t87-t165);
t480 = t263.*t447;
t484 = t291.*t447;
t492 = t5.*t305.*t447;
t493 = t11.*t305.*t447;
t494 = t313.*t447;
t497 = t345.*t447;
t500 = -t447.*(t198-t279);
t502 = t447.*(t198-t279);
t503 = t350.*t447;
t506 = -t447.*(t229+t11.*(t98-t169));
t508 = -t447.*(t207-t293);
t337 = -t326;
t361 = t242+t324;
t364 = t244+t336;
t370 = -t366;
t392 = t246+t323+t342;
t405 = t309.*t382;
t416 = t317+t318+t339;
t421 = ddy.*t417;
t423 = ddz.*t422;
t437 = t152+t189+t190+t297+t299+t302;
t444 = t305.*t415;
t449 = t27+t61+t153+t159+t191+t329+t330+t341;
t461 = -t458;
t465 = t415.*(t328-t5.*(t55-t150));
t467 = -t415.*(t325+t11.*(t55-t150));
t469 = t415.*(t325+t11.*(t55-t150));
t481 = -t480;
t486 = -t484;
t495 = -t492;
t504 = t352.*t447;
t507 = -t503;
t363 = t240+t337;
t365 = t4.*t6.*t361;
t374 = t133.*t361;
t376 = t142.*t361;
t395 = ddx.*t392;
t410 = -t405;
t424 = -t421;
t425 = -t423;
t436 = t361.*t382;
t445 = t309.*t416;
t453 = t305.*t437;
t459 = t361.*t407;
t463 = t361.*t416;
t468 = -t465;
t482 = t248.*t449;
t483 = t261.*t449;
t487 = -t361.*(-t137-t161+t188+T_fur_gap.*(t163-t180)+T_length.*(t163-t180).*(7.0./1.0e+1)+bar_len.*(t163-t180));
t489 = t437.*(t328-t5.*(t55-t150));
t490 = -t437.*(t325+t11.*(t55-t150));
t491 = -t449.*(t163-t180);
t496 = t311.*t449;
t498 = t5.*t309.*t449;
t499 = t11.*t309.*t449;
t505 = t344.*t449;
t509 = -t504;
t510 = t346.*t449;
t511 = t348.*t449;
t512 = -t449.*(t170-t294);
t513 = t449.*(t170-t294);
t514 = t359.*t449;
t515 = t360.*t449;
t367 = t4.*t6.*t363;
t368 = -t365;
t377 = t133.*t363;
t380 = t142.*t363;
t439 = t363.*t382;
t446 = -t445;
t454 = -ddx.*(t365+t12.*(t147-t245)+t6.*t10.*(t325+t11.*(t55-t150)));
t456 = -t453;
t457 = ddx.*(t365+t12.*(t147-t245)+t6.*t10.*(t325+t11.*(t55-t150)));
t462 = t363.*t407;
t466 = t363.*t416;
Q_added_tail_4_drag = ft_1({M_add,T_fur_gap,T_length,bar_len,ddphi1,ddphi2,ddth1,ddth2,ddx,ddy,ddz,t10,t11,t12,t132,t133,t134,t137,t141,t142,t147,t150,t161,t163,t165,t169,t171,t180,t183,t185,t188,t2,t207,t215,t220,t225,t227,t228,t229,t232,t245,t293,t30,t304,t305,t309,t311,t313,t314,t321,t325,t327,t328,t334,t335,t343,t355,t361,t363,t367,t368,t369,t370,t371,t372,t374,t375,t376,t377,t378,t379,t380,t381,t382,t384,t386,t387,t388,t389,t390,t391,t393,t394,t395,t396,t397,t398,t399,t4,t400,t401,t403,t404,t406,t407,t408,t409,t410,t411,t413,t414,t415,t416,t418,t419,t420,t424,t425,t426,t427,t428,t430,t431,t432,t433,t434,t436,t437,t438,t439,t440,t442,t443,t444,t445,t446,t447,t449,t452,t453,t454,t455,t456,t457,t458,t459,t461,t462,t463,t464,t465,t466,t468,t469,t479,t481,t482,t483,t484,t486,t487,t489,t490,t491,t493,t494,t495,t496,t497,t498,t499,t5,t502,t504,t505,t506,t507,t508,t509,t510,t511,t512,t513,t514,t515,t55,t6,t62,t69,t8,t87,t98,t99});
end
function Q_added_tail_4_drag = ft_1(ct)
M_add = ct{1};
T_fur_gap = ct{2};
T_length = ct{3};
bar_len = ct{4};
ddphi1 = ct{5};
ddphi2 = ct{6};
ddth1 = ct{7};
ddth2 = ct{8};
ddx = ct{9};
ddy = ct{10};
ddz = ct{11};
t10 = ct{12};
t11 = ct{13};
t12 = ct{14};
t132 = ct{15};
t133 = ct{16};
t134 = ct{17};
t137 = ct{18};
t141 = ct{19};
t142 = ct{20};
t147 = ct{21};
t150 = ct{22};
t161 = ct{23};
t163 = ct{24};
t165 = ct{25};
t169 = ct{26};
t171 = ct{27};
t180 = ct{28};
t183 = ct{29};
t185 = ct{30};
t188 = ct{31};
t2 = ct{32};
t207 = ct{33};
t215 = ct{34};
t220 = ct{35};
t225 = ct{36};
t227 = ct{37};
t228 = ct{38};
t229 = ct{39};
t232 = ct{40};
t245 = ct{41};
t293 = ct{42};
t30 = ct{43};
t304 = ct{44};
t305 = ct{45};
t309 = ct{46};
t311 = ct{47};
t313 = ct{48};
t314 = ct{49};
t321 = ct{50};
t325 = ct{51};
t327 = ct{52};
t328 = ct{53};
t334 = ct{54};
t335 = ct{55};
t343 = ct{56};
t355 = ct{57};
t361 = ct{58};
t363 = ct{59};
t367 = ct{60};
t368 = ct{61};
t369 = ct{62};
t370 = ct{63};
t371 = ct{64};
t372 = ct{65};
t374 = ct{66};
t375 = ct{67};
t376 = ct{68};
t377 = ct{69};
t378 = ct{70};
t379 = ct{71};
t380 = ct{72};
t381 = ct{73};
t382 = ct{74};
t384 = ct{75};
t386 = ct{76};
t387 = ct{77};
t388 = ct{78};
t389 = ct{79};
t390 = ct{80};
t391 = ct{81};
t393 = ct{82};
t394 = ct{83};
t395 = ct{84};
t396 = ct{85};
t397 = ct{86};
t398 = ct{87};
t399 = ct{88};
t4 = ct{89};
t400 = ct{90};
t401 = ct{91};
t403 = ct{92};
t404 = ct{93};
t406 = ct{94};
t407 = ct{95};
t408 = ct{96};
t409 = ct{97};
t410 = ct{98};
t411 = ct{99};
t413 = ct{100};
t414 = ct{101};
t415 = ct{102};
t416 = ct{103};
t418 = ct{104};
t419 = ct{105};
t420 = ct{106};
t424 = ct{107};
t425 = ct{108};
t426 = ct{109};
t427 = ct{110};
t428 = ct{111};
t430 = ct{112};
t431 = ct{113};
t432 = ct{114};
t433 = ct{115};
t434 = ct{116};
t436 = ct{117};
t437 = ct{118};
t438 = ct{119};
t439 = ct{120};
t440 = ct{121};
t442 = ct{122};
t443 = ct{123};
t444 = ct{124};
t445 = ct{125};
t446 = ct{126};
t447 = ct{127};
t449 = ct{128};
t452 = ct{129};
t453 = ct{130};
t454 = ct{131};
t455 = ct{132};
t456 = ct{133};
t457 = ct{134};
t458 = ct{135};
t459 = ct{136};
t461 = ct{137};
t462 = ct{138};
t463 = ct{139};
t464 = ct{140};
t465 = ct{141};
t466 = ct{142};
t468 = ct{143};
t469 = ct{144};
t479 = ct{145};
t481 = ct{146};
t482 = ct{147};
t483 = ct{148};
t484 = ct{149};
t486 = ct{150};
t487 = ct{151};
t489 = ct{152};
t490 = ct{153};
t491 = ct{154};
t493 = ct{155};
t494 = ct{156};
t495 = ct{157};
t496 = ct{158};
t497 = ct{159};
t498 = ct{160};
t499 = ct{161};
t5 = ct{162};
t502 = ct{163};
t504 = ct{164};
t505 = ct{165};
t506 = ct{166};
t507 = ct{167};
t508 = ct{168};
t509 = ct{169};
t510 = ct{170};
t511 = ct{171};
t512 = ct{172};
t513 = ct{173};
t514 = ct{174};
t515 = ct{175};
t55 = ct{176};
t6 = ct{177};
t62 = ct{178};
t69 = ct{179};
t8 = ct{180};
t87 = ct{181};
t98 = ct{182};
t99 = ct{183};
t471 = t334+t374+t381;
t474 = -ddy.*(-t374+t141.*(t325+t11.*(t55-t150))+t6.*t8.*(t147-t245));
t476 = t343+t376+t379;
t485 = -t483;
t488 = -t363.*(-t137-t161+t188+T_fur_gap.*(t163-t180)+T_length.*(t163-t180).*(7.0./1.0e+1)+bar_len.*(t163-t180));
t501 = -t499;
t516 = -t515;
t517 = t372+t401+t406+t410+t479+t482;
t522 = t386+t427+t436+t440+t507+t514;
t524 = -ddphi2.*(t387+t404-t444+t445-t494-t496);
t527 = ddphi2.*(t387+t404-t444+t445-t494-t496);
t529 = -ddphi1.*(-t400+t452+t453+t484+t225.*(t30+t62+t69-t183-t185-t220)+t449.*(t163-t180));
t532 = t396+t414+t463+t469+t495+t498;
t539 = t431+t433+t459+t464+t502+t510;
t543 = -ddphi1.*(-t489+t504-t511+t304.*(t30+t62+t69-t183-t185-t220)+t363.*(-t137-t161+t188+T_fur_gap.*(t163-t180)+T_length.*(t163-t180).*(7.0./1.0e+1)+bar_len.*(t163-t180))+t390.*(t99-t215));
t544 = t399+t420+t487+t490+t508+t513;
t545 = -ddphi1.*(t398+t418+t512+t437.*(t325+t11.*(t55-t150))+t361.*(-t137-t161+t188+T_fur_gap.*(t163-t180)+T_length.*(t163-t180).*(7.0./1.0e+1)+bar_len.*(t163-t180))+t447.*(t207-t293));
t448 = t314+t367+t370;
t451 = t327+t368+t369;
t470 = t321+t375+t380;
t472 = t335+t377+t378;
t478 = ddz.*t476;
t518 = ddth2.*t517;
t519 = t403+t411+t442+t443+t481+t485;
t521 = t389+t409+t444+t446+t494+t496;
t523 = t384+t428+t438+t439+t506+t516;
t525 = ddth2.*t522;
t526 = -ddth2.*(-t384+t426-t439+t515+t447.*(t229+t11.*(t98-t169))+(t328-t5.*(t55-t150)).*(T_fur_gap.*(t87-t165)+T_length.*(t87-t165).*(7.0./1.0e+1)+bar_len.*(t87-t165)));
t528 = t388+t400+t455+t456+t486+t491;
t530 = t397+t413+t466+t468+t493+t501;
t531 = -ddphi2.*(t393-t413+t465-t466-t493+t499);
t533 = ddphi2.*(t393-t413+t465-t466-t493+t499);
t534 = ddphi2.*t532;
t536 = t430+t434+t461+t462+t497+t505;
t537 = -ddth1.*(t432+t458-t462-t497-t505+t390.*(t171-t232));
t538 = ddth1.*(t432+t458-t462-t497-t505+t390.*(t171-t232));
t540 = ddth1.*t539;
t542 = t394+t419+t488+t489+t509+t511;
t450 = ddx.*t448;
t473 = ddz.*t470;
t475 = ddy.*t472;
t520 = ddth1.*t519;
t535 = -t534;
t541 = -t540;
t557 = -M_add.*t227.*(t454-t478-t525+t534+t540+ddy.*(-t374+t141.*(t325+t11.*(t55-t150))+t6.*t8.*(t147-t245))+ddphi1.*(t398+t418+t512+t437.*(t325+t11.*(t55-t150))+t361.*(-t137-t161+t188+T_fur_gap.*(t163-t180)+T_length.*(t163-t180).*(7.0./1.0e+1)+bar_len.*(t163-t180))+t447.*(t207-t293)));
t558 = M_add.*t227.*(t454-t478-t525+t534+t540+ddy.*(-t374+t141.*(t325+t11.*(t55-t150))+t6.*t8.*(t147-t245))+ddphi1.*(t398+t418+t512+t437.*(t325+t11.*(t55-t150))+t361.*(-t137-t161+t188+T_fur_gap.*(t163-t180)+T_length.*(t163-t180).*(7.0./1.0e+1)+bar_len.*(t163-t180))+t447.*(t207-t293)));
t559 = -M_add.*t311.*(t454-t478-t525+t534+t540+ddy.*(-t374+t141.*(t325+t11.*(t55-t150))+t6.*t8.*(t147-t245))+ddphi1.*(t398+t418+t512+t437.*(t325+t11.*(t55-t150))+t361.*(-t137-t161+t188+T_fur_gap.*(t163-t180)+T_length.*(t163-t180).*(7.0./1.0e+1)+bar_len.*(t163-t180))+t447.*(t207-t293)));
t560 = -M_add.*t313.*(t454-t478-t525+t534+t540+ddy.*(-t374+t141.*(t325+t11.*(t55-t150))+t6.*t8.*(t147-t245))+ddphi1.*(t398+t418+t512+t437.*(t325+t11.*(t55-t150))+t361.*(-t137-t161+t188+T_fur_gap.*(t163-t180)+T_length.*(t163-t180).*(7.0./1.0e+1)+bar_len.*(t163-t180))+t447.*(t207-t293)));
t546 = t395+t424+t425+t518+t520+t527+t529;
t551 = t450+t473+t475+t526+t533+t538+t543;
t553 = t457+t474+t478+t525+t535+t541+t545;
t547 = M_add.*t225.*t546;
t548 = M_add.*t305.*t546;
t549 = M_add.*t309.*t546;
t552 = M_add.*t132.*t551;
t554 = M_add.*t228.*t551;
t555 = -M_add.*t551.*(t55-t150);
t556 = M_add.*t551.*(t55-t150);
t550 = -t549;
t561 = t547+t552+t558;
t562 = t548+t556+t560;
t563 = t550+t554+t559;
mt1 = [-t12.*t561-t6.*t10.*t562+t4.*t6.*(t549-t554+M_add.*t311.*(t454-t478-t525+t534+t540+ddy.*(-t374+t141.*(t325+t11.*(t55-t150))+t6.*t8.*(t147-t245))+ddphi1.*(t398+t418+t512+t437.*(t325+t11.*(t55-t150))+t361.*(-t137-t161+t188+T_fur_gap.*(t163-t180)+T_length.*(t163-t180).*(7.0./1.0e+1)+bar_len.*(t163-t180))+t447.*(t207-t293))))];
mt2 = [t141.*t562+t133.*(t549-t554+M_add.*t311.*(t454-t478-t525+t534+t540+ddy.*(-t374+t141.*(t325+t11.*(t55-t150))+t6.*t8.*(t147-t245))+ddphi1.*(t398+t418+t512+t437.*(t325+t11.*(t55-t150))+t361.*(-t137-t161+t188+T_fur_gap.*(t163-t180)+T_length.*(t163-t180).*(7.0./1.0e+1)+bar_len.*(t163-t180))+t447.*(t207-t293))))+t6.*t8.*t561];
mt3 = [t134.*t562+t142.*(t549-t554+M_add.*t311.*(t454-t478-t525+t534+t540+ddy.*(-t374+t141.*(t325+t11.*(t55-t150))+t6.*t8.*(t147-t245))+ddphi1.*(t398+t418+t512+t437.*(t325+t11.*(t55-t150))+t361.*(-t137-t161+t188+T_fur_gap.*(t163-t180)+T_length.*(t163-t180).*(7.0./1.0e+1)+bar_len.*(t163-t180))+t447.*(t207-t293))))-t2.*t6.*t561];
mt4 = [t561.*(t30+t62+t69-t183-t185-t220)+t437.*t562-(t549-t554+M_add.*t311.*(t454-t478-t525+t534+t540+ddy.*(-t374+t141.*(t325+t11.*(t55-t150))+t6.*t8.*(t147-t245))+ddphi1.*(t398+t418+t512+t437.*(t325+t11.*(t55-t150))+t361.*(-t137-t161+t188+T_fur_gap.*(t163-t180)+T_length.*(t163-t180).*(7.0./1.0e+1)+bar_len.*(t163-t180))+t447.*(t207-t293)))).*(-t137-t161+t188+T_fur_gap.*(t163-t180)+T_length.*(t163-t180).*(7.0./1.0e+1)+bar_len.*(t163-t180))];
mt5 = [-t391.*t561+t408.*t562-t407.*(t549-t554+M_add.*t311.*(t454-t478-t525+t534+t540+ddy.*(-t374+t141.*(t325+t11.*(t55-t150))+t6.*t8.*(t147-t245))+ddphi1.*(t398+t418+t512+t437.*(t325+t11.*(t55-t150))+t361.*(-t137-t161+t188+T_fur_gap.*(t163-t180)+T_length.*(t163-t180).*(7.0./1.0e+1)+bar_len.*(t163-t180))+t447.*(t207-t293))))];
mt6 = [-t449.*t562-t447.*(t549-t554+M_add.*t311.*(t454-t478-t525+t534+t540+ddy.*(-t374+t141.*(t325+t11.*(t55-t150))+t6.*t8.*(t147-t245))+ddphi1.*(t398+t418+t512+t437.*(t325+t11.*(t55-t150))+t361.*(-t137-t161+t188+T_fur_gap.*(t163-t180)+T_length.*(t163-t180).*(7.0./1.0e+1)+bar_len.*(t163-t180))+t447.*(t207-t293))))];
mt7 = [-t371.*t561+t415.*t562-t416.*(t549-t554+M_add.*t311.*(t454-t478-t525+t534+t540+ddy.*(-t374+t141.*(t325+t11.*(t55-t150))+t6.*t8.*(t147-t245))+ddphi1.*(t398+t418+t512+t437.*(t325+t11.*(t55-t150))+t361.*(-t137-t161+t188+T_fur_gap.*(t163-t180)+T_length.*(t163-t180).*(7.0./1.0e+1)+bar_len.*(t163-t180))+t447.*(t207-t293))))];
mt8 = [-t355.*t561-t562.*(T_fur_gap.*(t87-t165)+T_length.*(t87-t165).*(7.0./1.0e+1)+bar_len.*(t87-t165))+t382.*(t549-t554+M_add.*t311.*(t454-t478-t525+t534+t540+ddy.*(-t374+t141.*(t325+t11.*(t55-t150))+t6.*t8.*(t147-t245))+ddphi1.*(t398+t418+t512+t437.*(t325+t11.*(t55-t150))+t361.*(-t137-t161+t188+T_fur_gap.*(t163-t180)+T_length.*(t163-t180).*(7.0./1.0e+1)+bar_len.*(t163-t180))+t447.*(t207-t293))))];
Q_added_tail_4_drag = [mt1;mt2;mt3;mt4;mt5;mt6;mt7;mt8];
end
